simulink model "MassSpring_Simulink"  (R2016b)
settings: Solver=VariableStepAuto  StartTime=0.0  StopTime=10.0  RelTol=1e-3
settings Model: Creator=ixohoxi  LastModifiedBy=ixohoxi

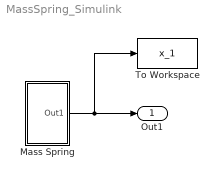
== system MassSpring_Simulink ==
  Mass Spring : Subsystem  mask{x_e=0.5, alpha=pi/6, mu=0.1, g=9.8, m=1, k=3}
      mask prompts: x_e "spring equilibrium"; alpha "incline angle"; mu "coefficient friction"; g "gravitation"; m "mass"; k "spring cont"
  To Workspace : ToWorkspace  VariableName=x_1  SaveFormat=Timeseries  SampleTime=-1
  Out1 : Outport
  wires:
  Mass Spring/1(Out1) -> To Workspace/1, Out1/1

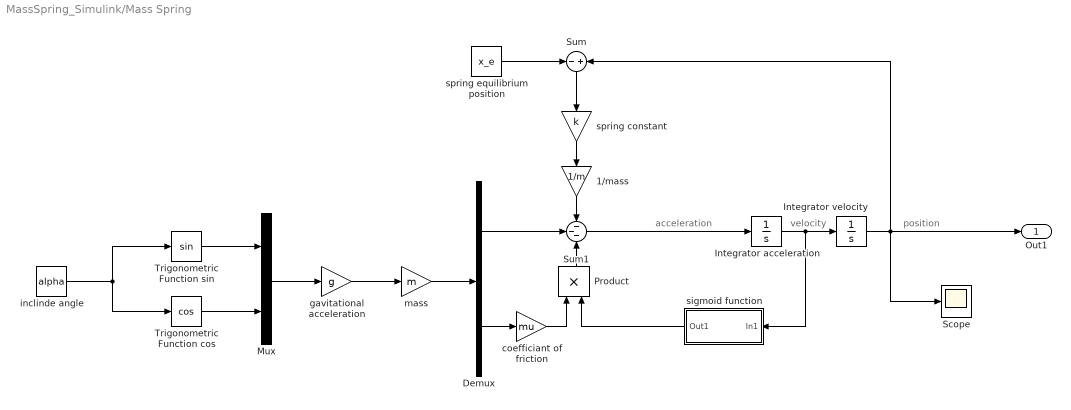
== system MassSpring_Simulink/Mass Spring ==
  note: acceleration
  note: velocity
  note: position
  "1/mass " : Gain  Gain=1/m
  Demux : Demux  Outputs=2
  Integrator acceleration : Integrator
  "Integrator velocity " : Integrator
  Mux : Mux  Inputs=2
  Product : Product
  Scope : Scope
  Sum : Sum  Inputs=-+
  Sum1 : Sum  Inputs=---
  Trigonometric Function cos : Trigonometry  Operator=cos
  Trigonometric Function sin : Trigonometry
  coefficiant of friction : Gain  Gain=mu
  gavitational acceleration : Gain  Gain=g
  inclinde angle : Constant  Value=alpha
  mass : Gain  Gain=m
  sigmoid function : Subsystem  mask{a=20}
      mask prompts: a "growth factor"
  spring constant : Gain  Gain=k
  "spring equilibrium position " : Constant  Value=x_e
  Out1 : Outport
  wires:
  sigmoid function/1(Out1) -> Product/2
  "spring equilibrium position "/1 -> Sum/1
  Integrator acceleration/1 -> sigmoid function/1(In1), "Integrator velocity "/1
  spring constant/1 -> "1/mass "/1
  "1/mass "/1 -> Sum1/1
  mass/1 -> Demux/1
  Demux/2 -> coefficiant of friction/1
  inclinde angle/1 -> Trigonometric Function cos/1, Trigonometric Function sin/1
  Trigonometric Function cos/1 -> Mux/2
  Mux/1 -> gavitational acceleration/1
  Trigonometric Function sin/1 -> Mux/1
  "Integrator velocity "/1 -> Out1/1, Scope/1, Sum/2
  gavitational acceleration/1 -> mass/1
  Product/1 -> Sum1/3
  Demux/1 -> Sum1/2
  coefficiant of friction/1 -> Product/1
  Sum1/1 -> Integrator acceleration/1
  Sum/1 -> spring constant/1

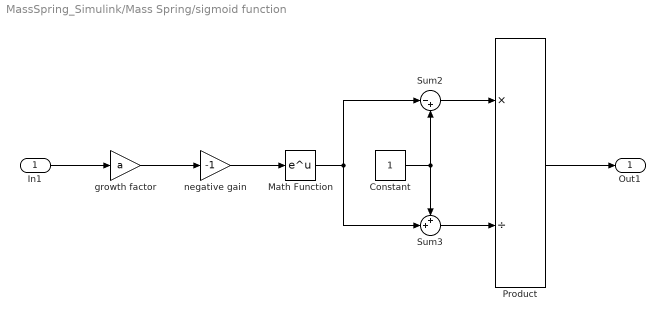
== system MassSpring_Simulink/Mass Spring/sigmoid function ==
  In1 : Inport
  Constant : Constant
  Math Function : Math  SaturateOnIntegerOverflow=on
  Product : Product  Inputs=*/
  Sum2 : Sum  Inputs=|-+
  Sum3 : Sum  Inputs=++|
  growth factor : Gain  Gain=a
  negative gain : Gain  Gain=-1
  Out1 : Outport
  wires:
  Sum2/1 -> Product/1
  Math Function/1 -> Sum3/2, Sum2/1
  Product/1 -> Out1/1
  Sum3/1 -> Product/2
  Constant/1 -> Sum3/1, Sum2/2
  In1/1 -> growth factor/1
  growth factor/1 -> negative gain/1
  negative gain/1 -> Math Function/1
